simulink model "sampleModel1633"  (R2023a)
settings: Solver=VariableStepAuto  StartTime=0.0  StopTime=10.0  RelTol=1e-3
libraries: hdlsllib x5, simulink x2
settings Model: Creator=user1  LastModifiedBy=user1

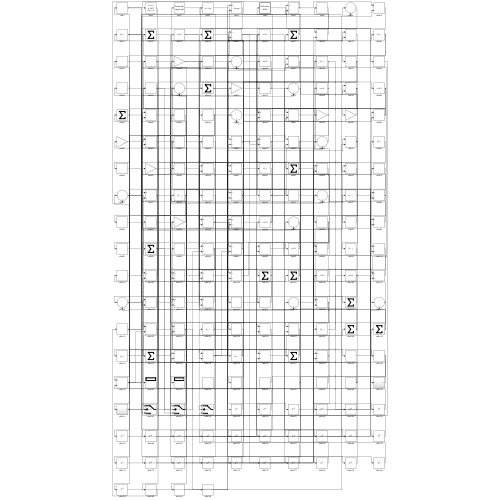
[thumbnail: Simulink's stored preview of the top-level diagram]
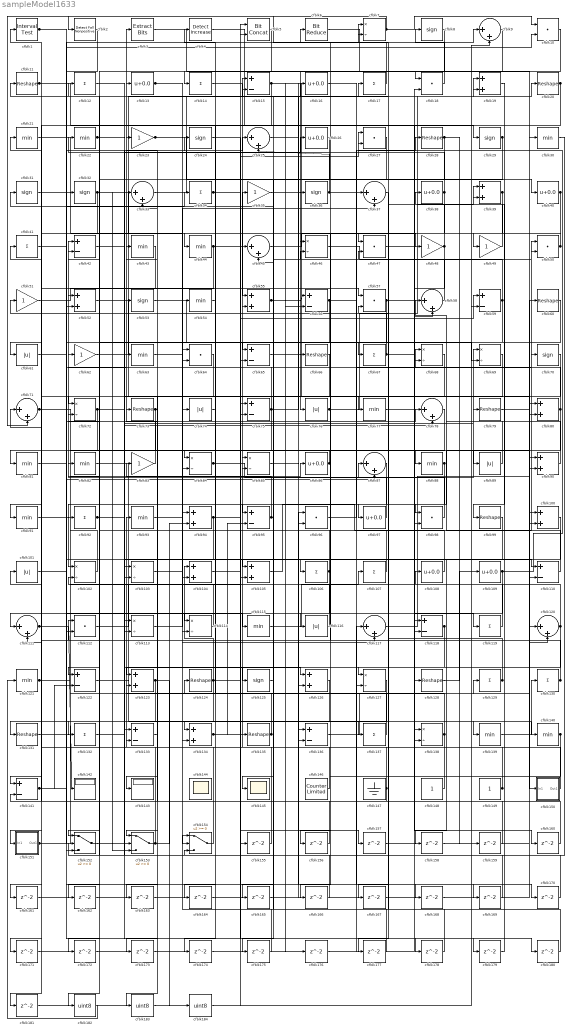
== system sampleModel1633 ==
  cfblk1 : hdlsllib/Logic and Bit Operations/Interval Test  IntervalClosedRight=on  uplimit=0.5  IntervalClosedLeft=on  lowlimit=-0.5  OutDataTypeStr=boolean
  cfblk{10,18,27,47,50,57,64,96,98,112} (10 alike) : DotProduct  OutDataTypeStr=Inherit: Inherit via internal rule
  cfblk{19,39,52,55,80,90,94,100,104..105,123,126,134} (13 alike) : Sum
  cfblk{61,74,76,89,101,116} (6 alike) : Abs  SaturateOnIntegerOverflow=off
  cfblk{7,46,68..69,72,84..85,102..103,113..114,127,138} (13 alike) : Product  Inputs=*/  RndMeth=Zero  SaturateOnIntegerOverflow=on
  cfblk{12,14,17,34,41,67,92,106..107,119,129..130,132,137} (14 alike) : Sum  Inputs=+
  cfblk{13,16,26,38,40,86,97,108..109} (9 alike) : Bias  Bias=0.0  SaturateOnIntegerOverflow=off
  cfblk{11,20,28,60,66,73,79,99,124,128,131,135} (12 alike) : Reshape
  cfblk{15,42,56,59,65,75,95,110,118,122,133,136,141} (13 alike) : Sum  Inputs=+-
  cfblk{9,25,33,37,45,58,71,78,87,111,117,120} (12 alike) : Sum  Inputs=|++
  cfblk{21..22,30,43..44,54,63,77,81..82,88,91,93,115,121,139..140} (17 alike) : MinMax
  cfblk{8,24,29,31..32,36,53,70,125} (9 alike) : Signum
  cfblk142 : Display
  cfblk143 : Display
  cfblk144 : Scope
      settings: Floating=on
  cfblk145 : Scope
  cfblk146 : hdlsllib/Sources/Counter Limited  uplimit=7  tsamp=-1
  cfblk147 : Ground
  cfblk148 : Constant  SampleTime=-1
  cfblk149 : Constant  SampleTime=-1
  cfblk150 : Subsystem
      settings: LibrarySourceBlock=|
      | hdlsllib/Ports &
      | Subsystems/Subsystem
  cfblk151 : Subsystem
      settings: LibrarySourceBlock=|
      | hdlsllib/Ports &
      | Subsystems/Subsystem
  cfblk152 : Switch  SaturateOnIntegerOverflow=off  InputSameDT=off
  cfblk153 : Switch  SaturateOnIntegerOverflow=off  InputSameDT=off
  cfblk154 : Switch  SaturateOnIntegerOverflow=off  InputSameDT=off
  cfblk{155..181} (27 alike) : Delay  SampleTime=1
  cfblk182 : DataTypeConversion  OutDataTypeStr=uint8  SaturateOnIntegerOverflow=off  RndMeth=Floor
  cfblk183 : DataTypeConversion  OutDataTypeStr=uint8  SaturateOnIntegerOverflow=off  RndMeth=Floor
  cfblk184 : DataTypeConversion  OutDataTypeStr=uint8  SaturateOnIntegerOverflow=off  RndMeth=Floor
  cfblk2 : hdlsllib/Logic and Bit Operations/Detect Fall Nonpositive  vinit=0  OutDataTypeStr=boolean
  cfblk{23,35,48..49,51,62,83} (7 alike) : Gain
  cfblk3 : simulink/Logic and Bit Operations/Extract Bits  bitsToExtract=Upper half  numBits=8  bitIdxRange=[0 7]  outScalingMode=Preserve fixed-point scaling
      settings: LibrarySourceBlock=|
      | hdlsllib/Logic and Bit
      | Operations/Extract Bits
  cfblk4 : simulink/Logic and Bit Operations/Detect Increase  vinit=0.0  OutDataTypeStr=boolean
      settings: LibrarySourceBlock=|
      | hdlsllib/Logic and Bit
      | Operations/Detect
      | Increase
  cfblk5 : hdlsllib/Logic and Bit Operations/Bit Concat  numInputs=2
  cfblk6 : hdlsllib/Logic and Bit Operations/Bit Reduce  mode=AND
  wires:
  cfblk65/1 -> cfblk76/1
  cfblk4/1 -> cfblk29/1
  cfblk82/1 -> cfblk139/1
  cfblk146/1 -> cfblk93/1
  cfblk124/1 -> cfblk104/1, cfblk86/1, cfblk181/1
  cfblk17/1 -> cfblk71/2
  cfblk14/1 -> cfblk57/1
  cfblk102/1 -> cfblk88/1
  cfblk66/1 -> cfblk153/1
  cfblk83/1 -> cfblk3/1
  cfblk128/1 -> cfblk109/1
  cfblk84/1 -> cfblk69/1, cfblk126/2
  cfblk97/1 -> cfblk42/1
  cfblk113/1 -> cfblk64/1
  cfblk88/1 -> cfblk97/1, cfblk122/1
  cfblk105/1 -> cfblk50/1
  cfblk67/1 -> cfblk51/1, cfblk119/1
  cfblk109/1 -> cfblk27/1, cfblk116/1
  cfblk62/1 -> cfblk17/1
  cfblk18/1 -> cfblk8/1
  cfblk74/1 -> cfblk114/1
  cfblk60/1 -> cfblk127/1
  cfblk15/1 -> cfblk150/1(In1), cfblk67/1, cfblk111/2, cfblk176/1
  cfblk154/1 -> cfblk43/1
  cfblk8/1 -> cfblk14/1
  cfblk115/1 -> cfblk107/1
  cfblk140/1 -> cfblk166/1, cfblk167/1
  cfblk90/1 -> cfblk62/1
  cfblk117/1 -> cfblk60/1
  cfblk92/1 -> cfblk79/1, cfblk153/3
  cfblk153/1 -> cfblk41/1, cfblk94/2
  cfblk57/1 -> cfblk39/1, cfblk72/1
  cfblk78/1 -> cfblk84/1
  cfblk56/1 -> cfblk37/1, cfblk75/2
  cfblk33/1 -> cfblk20/1
  cfblk149/1 -> cfblk35/1, cfblk47/2
  cfblk89/1 -> cfblk68/1
  cfblk121/1 -> cfblk85/1, cfblk63/1
  cfblk150/1(Out1) -> cfblk21/1
  cfblk22/1 -> cfblk126/1, cfblk172/1
  cfblk64/1 -> cfblk111/1
  cfblk3/1 -> cfblk30/1
  cfblk91/1 -> cfblk102/1
  cfblk49/1 -> cfblk11/1
  cfblk70/1 -> cfblk89/1
  cfblk123/1 -> cfblk23/1, cfblk141/1, cfblk184/1
  cfblk19/1 -> cfblk99/1
  cfblk151/1(Out1) -> cfblk129/1, cfblk78/1
  cfblk32/1 -> cfblk74/1, cfblk112/2, cfblk153/2
  cfblk43/1 -> cfblk61/1
  cfblk21/1 -> cfblk103/1
  cfblk147/1 -> cfblk33/1, cfblk141/2
  cfblk139/1 -> cfblk130/1
  cfblk120/1 -> cfblk138/2, cfblk15/1
  cfblk27/1 -> cfblk92/1
  cfblk38/1 -> cfblk22/1, cfblk46/1
  cfblk20/1 -> cfblk84/2, cfblk134/1
  cfblk11/1 -> cfblk118/1, cfblk69/2, cfblk10/2
  cfblk116/1 -> cfblk73/1
  cfblk9/1 -> cfblk18/1
  cfblk51/1 -> cfblk55/1
  cfblk7/1 -> cfblk2/1, cfblk10/1
  cfblk41/1 -> cfblk115/1
  cfblk100/1 -> cfblk103/2
  cfblk136/1 -> cfblk90/1
  cfblk94/1 -> cfblk143/1, cfblk134/2, cfblk157/1
  cfblk58/1 -> cfblk13/1
  cfblk98/1 -> cfblk87/1
  cfblk23/1 -> cfblk40/1, cfblk65/2
  cfblk96/1 -> cfblk70/1
  cfblk6/1 -> cfblk100/1
  cfblk13/1 -> cfblk104/2, cfblk117/2
  cfblk53/1 -> cfblk135/1
  cfblk29/1 -> cfblk105/1, cfblk175/1
  cfblk59/1 -> cfblk31/1, cfblk113/2
  cfblk112/1 -> cfblk45/1
  cfblk111/1 -> cfblk142/1, cfblk7/1
  cfblk85/1 -> cfblk136/1
  cfblk114/1 -> cfblk82/1
  cfblk130/1 -> cfblk6/1, cfblk101/1
  cfblk76/1 -> cfblk19/1, cfblk28/1
  cfblk73/1 -> cfblk152/1, cfblk33/2
  cfblk50/1 -> cfblk44/1, cfblk49/1
  cfblk110/1 -> cfblk58/1
  cfblk52/1 -> cfblk94/1
  cfblk69/1 -> cfblk125/1
  cfblk35/1 -> cfblk66/1
  cfblk34/1 -> cfblk90/2, cfblk27/2
  cfblk134/1 -> cfblk59/1, cfblk16/1, cfblk95/2
  cfblk87/1 -> cfblk96/2
  cfblk39/1 -> cfblk91/1, cfblk95/1
  cfblk26/1 -> cfblk65/1
  cfblk101/1 -> cfblk25/1
  cfblk36/1 -> cfblk140/1, cfblk25/2
  cfblk42/1 -> cfblk80/2
  cfblk80/1 -> cfblk98/1, cfblk15/2
  cfblk131/1 -> cfblk54/1
  cfblk93/1 -> cfblk37/2
  cfblk46/1 -> cfblk50/2
  cfblk1/1 -> cfblk110/1, cfblk87/2
  cfblk135/1 -> cfblk131/1, cfblk4/1
  cfblk10/1 -> cfblk36/1
  cfblk118/1 -> cfblk163/1, cfblk164/1
  cfblk122/1 -> cfblk137/1
  cfblk129/1 -> cfblk112/1, cfblk7/2
  cfblk30/1 -> cfblk152/2
  cfblk119/1 -> cfblk108/1
  cfblk40/1 -> cfblk47/1, cfblk156/1
  cfblk103/1 -> cfblk64/2
  cfblk63/1 -> cfblk106/1
  cfblk47/1 -> cfblk128/1
  cfblk68/1 -> cfblk123/1
  cfblk28/1 -> cfblk105/2, cfblk159/1
  cfblk61/1 -> cfblk9/1
  cfblk95/1 -> cfblk145/1, cfblk83/1
  cfblk86/1 -> cfblk81/1, cfblk46/2
  cfblk138/1 -> cfblk133/2, cfblk53/1
  cfblk72/1 -> cfblk151/1(In1), cfblk78/2
  cfblk31/1 -> cfblk114/2
  cfblk132/1 -> cfblk24/1
  cfblk81/1 -> cfblk34/1
  cfblk45/1 -> cfblk48/1
  cfblk55/1 -> cfblk56/1, cfblk56/2
  cfblk48/1 -> cfblk118/2, cfblk38/1
  cfblk137/1 -> cfblk124/1
  cfblk127/1 -> cfblk154/2
  cfblk148/1 -> cfblk52/1
  cfblk108/1 -> cfblk85/2
  cfblk71/1 -> cfblk52/2, cfblk113/1, cfblk170/1
  cfblk107/1 -> cfblk45/2
  cfblk2/1 -> cfblk152/3
  cfblk75/1 -> cfblk19/2, cfblk12/1, cfblk132/1
  cfblk106/1 -> cfblk72/2, cfblk171/1
  cfblk79/1 -> cfblk120/1
  cfblk141/1 -> cfblk32/1, cfblk122/2, cfblk180/1
  cfblk152/1 -> cfblk26/1
  cfblk44/1 -> cfblk77/1, cfblk161/1, cfblk162/1
  cfblk104/1 -> cfblk155/1
  cfblk155/1 -> cfblk1/1
  cfblk156/1 -> cfblk102/2
  cfblk157/1 -> cfblk110/2
  cfblk99/1 -> cfblk158/1
  cfblk158/1 -> cfblk80/1
  cfblk159/1 -> cfblk123/2
  cfblk77/1 -> cfblk160/1
  cfblk160/1 -> cfblk71/1
  cfblk161/1 -> cfblk136/2
  cfblk162/1 -> cfblk117/1
  cfblk163/1 -> cfblk100/2
  cfblk164/1 -> cfblk120/2
  cfblk125/1 -> cfblk165/1
  cfblk165/1 -> cfblk96/1
  cfblk166/1 -> cfblk42/2
  cfblk167/1 -> cfblk18/2
  cfblk25/1 -> cfblk168/1
  cfblk168/1 -> cfblk59/2
  cfblk16/1 -> cfblk169/1
  cfblk169/1 -> cfblk133/1
  cfblk170/1 -> cfblk154/3
  cfblk171/1 -> cfblk127/2
  cfblk172/1 -> cfblk138/1
  cfblk126/1 -> cfblk173/1
  cfblk173/1 -> cfblk68/2
  cfblk54/1 -> cfblk174/1
  cfblk174/1 -> cfblk58/2
  cfblk175/1 -> cfblk154/1
  cfblk176/1 -> cfblk98/2
  cfblk37/1 -> cfblk177/1
  cfblk177/1 -> cfblk55/2
  cfblk12/1 -> cfblk178/1
  cfblk178/1 -> cfblk75/1
  cfblk24/1 -> cfblk179/1
  cfblk179/1 -> cfblk39/2
  cfblk180/1 -> cfblk57/2
  cfblk181/1 -> cfblk9/2
  cfblk5/1 -> cfblk182/1
  cfblk182/1 -> cfblk121/1
  cfblk133/1 -> cfblk183/1
  cfblk183/1 -> cfblk5/1
  cfblk184/1 -> cfblk5/2

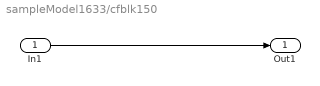
== system sampleModel1633/cfblk150 ==
  In1 : Inport
  Out1 : Outport
  wires:
  In1/1 -> Out1/1

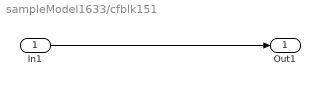
== system sampleModel1633/cfblk151 ==
  In1 : Inport
  Out1 : Outport
  wires:
  In1/1 -> Out1/1
